simulink model "mcb_pmsm_foc_host_model_dyno"  (R2024b)
settings: Solver=FixedStepDiscrete  StartTime=0.0  StopTime=inf  RelTol=1e-3  EnableMultiTasking=on
values from neighbouring files (symbols this model uses):
  dataType = 'single'    [mcb_pmsm_foc_dyno_f28379d_data.m]
  PU_System_motor1 = mcb_SetPUSystem(pmsm_motor1,inverter_motor1)    [mcb_pmsm_foc_dyno_f28379d_data.m]
  PU_System_motor2 = mcb_SetPUSystem(pmsm_motor2,inverter_motor2)    [mcb_pmsm_foc_dyno_f28379d_data.m]
  Ts = T_pwm    (= 5e-05)    [mcb_pmsm_foc_dyno_f28379d_data.m]
libraries: instrumentseriallib x4, simulink x3
settings Model: Creator=The MathWorks, Inc.  LastModifiedBy=giova
settings SolverCC: AlgebraicLoopSolver=TrustRegion  MaxZcPerStep=1
settings DataIOCC: LimitDataPoints=on  SaveFormat=Array  ReturnWorkspaceOutputs=off
settings OptimizationCC: ReuseModelBlockBuffer=off  LifeSpan=1  EfficientTunableParamExpr=on
settings DebuggingCC: UnderspecifiedInitializationDetection=Classic  MergeDetectMultiDrivingBlocksExec=none  SolverPrmCheckMsg=warning  ParameterPrecisionLossMsg=none  UnconnectedInputMsg=warning  UnconnectedOutputMsg=warning  UnconnectedLineMsg=warning  AllowSymbolicDim=off  PregeneratedLibrarySubsystemCodeDiagnostic=none  SubsystemReferenceDiagnosticForUnitTest=warning  SFUnexpectedBacktrackingDiag=warning  SFNoUnconditionalDefaultTransitionDiag=warning  SFExecutionAtInitializationDiag=none  ArithmeticOperatorsInVariantConditions=warning
settings HardwareCC: ProdBitPerPointer=32  ProdLargestAtomicFloat=None  ProdIntDivRoundTo=Undefined  ProdEndianess=Unspecified  ProdWordSize=32  ProdHWDeviceType=32-bit Generic
settings ModelReferenceCC: EnableRefExpFcnMdlSchedulingChecks=on  PropagateSignalLabelsOutOfModel=off
settings SFSimCC: SimUseLocalCustomCode=off  MATLABDynamicMemAlloc=off
settings RTWCC: Description=Real-Time Workshop Embedded Coder  SystemTargetFile=ert.tlc  TemplateMakefile=ert_default_tmf  GenerateReport=on  RTWUseLocalCustomCode=off  IncludeHyperlinkInReport=on  LaunchReport=on  GenerateTraceInfo=on  GenerateTraceReport=on  GenerateTraceReportSl=on  GenerateTraceReportSf=on  GenerateTraceReportEml=on  GPUComputeCapability=3.5  DLArmComputeVersion=19.05
settings CodeAppCC: IgnoreCustomStorageClasses=off  StateflowObjectComments=on  InternalIdentifier=Classic
settings ERTTargetCC: MultiwordLength=2048  GenerateSampleERTMain=on  InlinedParameterPlacement=Hierarchical  ERTCustomFileTemplate=example_file_process.tlc  ConvertIfToSwitch=off  SuppressUnreachableDefaultCases=off  DynamicArrayContainerType=coder::array
settings ConfigComp: CovMetricSettings=dw  CovSaveCumulativeToWorkspaceVar=on  CovSaveSingleToWorkspaceVar=on  CovExternalEMLEnable=off  CovSFcnEnable=off

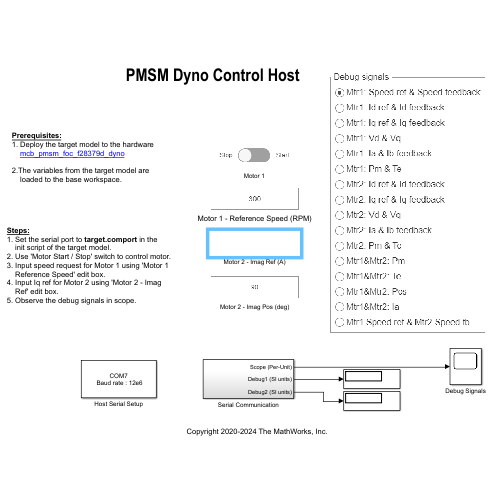
[thumbnail: Simulink's stored preview of the top-level diagram]
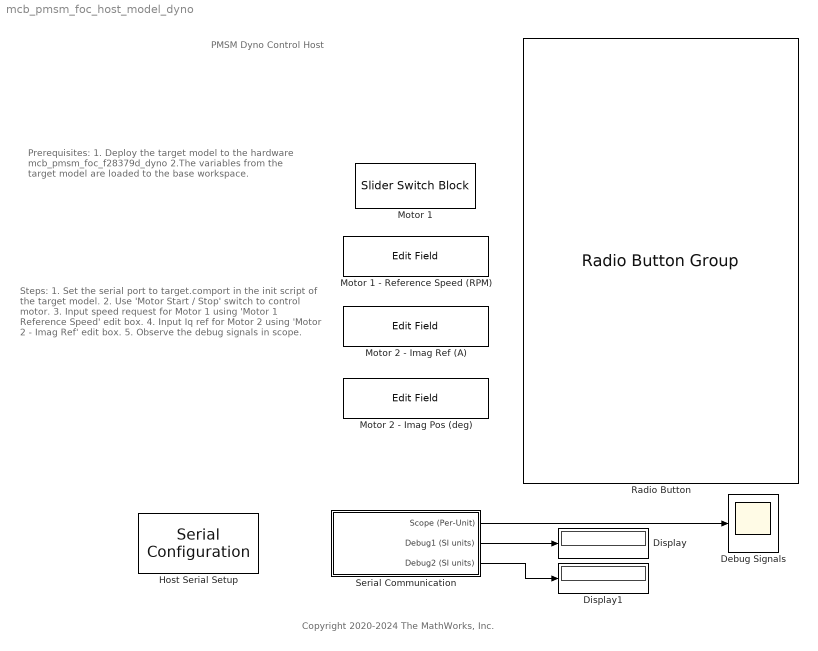
== system mcb_pmsm_foc_host_model_dyno ==
  note: PMSM Dyno Control Host
  note: Copyright 2020-2024 The MathWorks, Inc.
  note: Steps:
      | 1. Set the serial port to target.comport in the
      | init script of the target model.
      | 2. Use 'Motor Start / Stop' switch to control motor.
      | 3. Input speed request for Motor 1 using 'Motor 1
      | Reference Speed' edit box.
      | 4. Input Iq ref for Motor 2 using 'Motor 2 - Imag
      | Ref' edit box.
      | 5. Observe the debug signals in scope.
  note: Prerequisites:
      | 1. Deploy the target model to the hardware
      | mcb_pmsm_foc_f28379d_dyno
      |
      | 2.The variables from the target model are
      | loaded to the base workspace.
  Debug Signals : Scope
  Display : Display
  Display1 : Display
  Host Serial Setup : instrumentseriallib/Serial Configuration  Priority=-99  PortSel=COM7  Port=COM7  ComPort=COM7  BaudRate=12e6  DataBits=8  Parity=none  StopBits=1  ByteOrder=little-endian  FlowControl=none  Timeout=2  SimulateUsing=Interpreted execution  BlockInModel=on  aMode=5
      settings: LibrarySourceBlock=mcblib/Protection and Diagnostics/Host Serial Setup
  Motor 1 : SliderSwitchBlock  LabelPosition=Hide
      settings: Values={{'Stop', 'Start'}, [0 1]}
  Motor 1 - Reference Speed (RPM) : EditField  LabelPosition=Hide  ShowInitialText=on  Alignment=Center
  Motor 2 - Imag Pos (deg) : EditField  LabelPosition=Hide  ShowInitialText=on  Alignment=Center
  Motor 2 - Imag Ref (A) : EditField  LabelPosition=Hide  ShowInitialText=on  Alignment=Center
  Radio Button : RadioButtonGroup  LabelPosition=Hide  SelectedLabel=Mtr1: Speed ref & Speed feedback  ButtonGroupName=Debug signals
      settings: Values={{'Mtr1: Speed ref & Speed feedback', 'Mtr1: Id ref & Id feedback', 'Mtr1: Iq ref & Iq feedback', 'Mtr1: Vd & Vq', 'Mtr1: Ia & Ib feedback', 'Mtr1: Pm & Te', 'Mtr2: Id ref & Id feedback', 'Mtr2: Iq ref & Iq feedback', 'Mtr2: Vd & Vq', 'Mtr2: Ia & Ib feedback', 'Mtr2: Pm & Te', 'Mtr1&Mtr2: Pm', 'Mtr1&Mtr2: Te', 'Mtr1&Mtr2: Pos', 'Mtr1&Mtr2: Ia', 'Mtr1 Speed ref & Mtr2 Speed fb'}, [1 2 3 4 5 6 7 8 9 10 11 12 13 14 15 0]}
  Serial Communication : Subsystem
  wires:
  Serial Communication/1(Scope (Per-Unit)) -> Debug Signals/1
  Serial Communication/2(Debug1 (SI units)) -> Display/1
  Serial Communication/3(Debug2 (SI units)) -> Display1/1

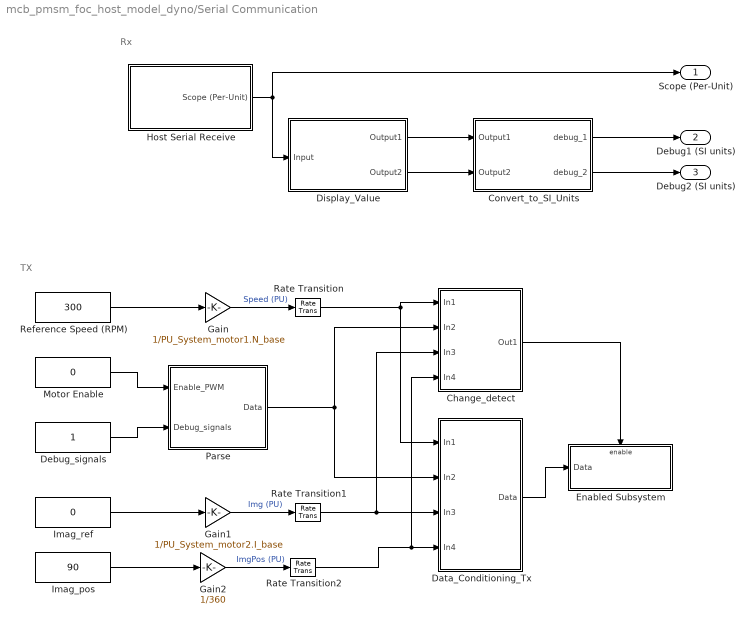
== system mcb_pmsm_foc_host_model_dyno/Serial Communication ==
  note: Rx
  note: TX
  Change_detect : Subsystem
  Convert_to_SI_Units : Subsystem
  Data_Conditioning_Tx : Subsystem  Variant=on
  Debug_signals : Constant  OutDataTypeStr=uint16  SampleTime=0.03
  Display_Value : MATLAB Function  TreatAsAtomicUnit=on
  Enabled Subsystem : Subsystem  TreatAsAtomicUnit=on
  Gain : Gain  Gain=1/PU_System_motor1.N_base  RndMeth=Simplest  OutDataTypeStr=Inherit: Same as input
  Gain1 : Gain  Gain=1/PU_System_motor2.I_base  RndMeth=Simplest  OutDataTypeStr=Inherit: Same as input
  Gain2 : Gain  Gain=1/360  RndMeth=Simplest  OutDataTypeStr=Inherit: Same as input
  Host Serial Receive : Subsystem  Variant=on
  Imag_pos : Constant  Value=90  VectorParams1D=off  OutDataTypeStr=single  SampleTime=0.03
  Imag_ref : Constant  Value=0  VectorParams1D=off  OutDataTypeStr=single  SampleTime=0.03
  Motor Enable : Constant  Value=0  VectorParams1D=off  OutDataTypeStr=uint16  SampleTime=0.03
  Parse : Subsystem
  Rate Transition : RateTransition  OutPortSampleTime=0.03
  Rate Transition1 : RateTransition  OutPortSampleTime=0.03
  Rate Transition2 : RateTransition  OutPortSampleTime=0.03
  Reference Speed (RPM) : Constant  Value=300  VectorParams1D=off  OutDataTypeStr=single  SampleTime=0.03
  Scope (Per-Unit) : Outport
  Debug1 (SI units) : Outport  Port=2
  Debug2 (SI units) : Outport  Port=3
  wires:
  Rate Transition2/1 -> Change_detect/4(In4), Data_Conditioning_Tx/4(In4)
  Imag_pos/1 -> Gain2/1
  Gain2/1 -> Rate Transition2/1  "ImgPos (PU)"
  Gain1/1 -> Rate Transition1/1  "Img (PU)"
  Rate Transition1/1 -> Change_detect/3(In3), Data_Conditioning_Tx/3(In3)
  Imag_ref/1 -> Gain1/1
  Motor Enable/1 -> Parse/1(Enable_PWM)
  Change_detect/1(Out1) -> Enabled Subsystem/Enable
  Reference Speed (RPM)/1 -> Gain/1
  Rate Transition/1 -> Data_Conditioning_Tx/1(In1), Change_detect/1(In1)
  Parse/1(Data) -> Change_detect/2(In2), Data_Conditioning_Tx/2(In2)
  Data_Conditioning_Tx/1(Data) -> Enabled Subsystem/1(Data)
  Gain/1 -> Rate Transition/1  "Speed (PU)"
  Debug_signals/1 -> Parse/2(Debug_signals)
  Convert_to_SI_Units/2(debug_2) -> Debug2 (SI units)/1
  Convert_to_SI_Units/1(debug_1) -> Debug1 (SI units)/1
  Host Serial Receive/1(Scope (Per-Unit)) -> Scope (Per-Unit)/1, Display_Value/1(Input)
  Display_Value/2(Output2) -> Convert_to_SI_Units/2(Output2)
  Display_Value/1(Output1) -> Convert_to_SI_Units/1(Output1)

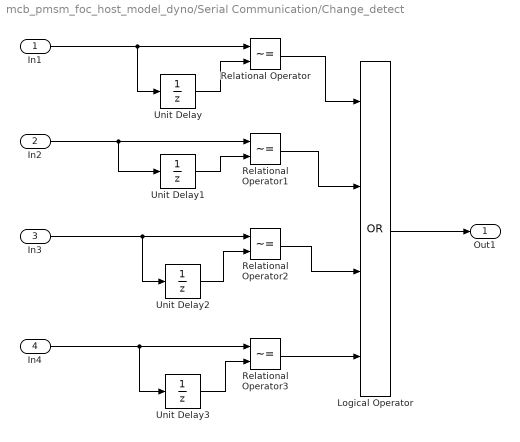
== system mcb_pmsm_foc_host_model_dyno/Serial Communication/Change_detect ==
  In1 : Inport
  In2 : Inport  Port=2
  In3 : Inport  Port=3
  In4 : Inport  Port=4
  Logical Operator : Logic  Operator=OR  Inputs=4  AllPortsSameDT=off  OutDataTypeStr=boolean
  Relational Operator{,1..3} (4 alike) : RelationalOperator  Operator=~=  OutDataTypeStr=boolean  InputSameDT=off
  Unit Delay : UnitDelay  InitialCondition=0.5  SampleTime=-1  HasFrameUpgradeWarning=on
  Unit Delay1 : UnitDelay  SampleTime=-1  HasFrameUpgradeWarning=on
  Unit Delay2 : UnitDelay  InitialCondition=0.5  SampleTime=-1  HasFrameUpgradeWarning=on
  Unit Delay3 : UnitDelay  InitialCondition=0.5  SampleTime=-1  HasFrameUpgradeWarning=on
  Out1 : Outport  VectorParamsAs1DForOutWhenUnconnected=off
  wires:
  In2/1 -> Relational Operator1/1, Unit Delay1/1
  Relational Operator1/1 -> Logical Operator/2
  Unit Delay1/1 -> Relational Operator1/2
  Unit Delay/1 -> Relational Operator/2
  In1/1 -> Unit Delay/1, Relational Operator/1
  Relational Operator/1 -> Logical Operator/1
  Logical Operator/1 -> Out1/1
  Relational Operator2/1 -> Logical Operator/3
  Unit Delay2/1 -> Relational Operator2/2
  In3/1 -> Unit Delay2/1, Relational Operator2/1
  In4/1 -> Unit Delay3/1, Relational Operator3/1
  Unit Delay3/1 -> Relational Operator3/2
  Relational Operator3/1 -> Logical Operator/4

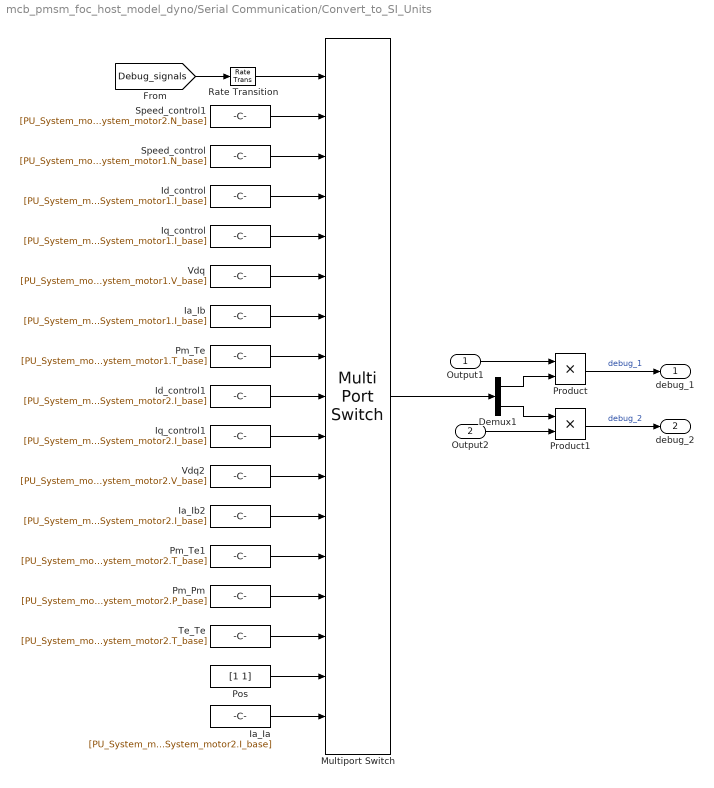
== system mcb_pmsm_foc_host_model_dyno/Serial Communication/Convert_to_SI_Units ==
  Output1 : Inport
  Output2 : Inport  Port=2
  Demux1 : Demux  Outputs=2
  Ia_Ia : Constant  Value=[PU_System_motor1.I_base PU_System_motor2.I_base]  OutDataTypeStr=single  SampleTime=-1
  Ia_Ib : Constant  Value=[PU_System_motor1.I_base PU_System_motor1.I_base]  OutDataTypeStr=single  SampleTime=-1
  Ia_Ib2 : Constant  Value=[PU_System_motor2.I_base PU_System_motor2.I_base]  OutDataTypeStr=single  SampleTime=-1
  Id_control : Constant  Value=[PU_System_motor1.I_base PU_System_motor1.I_base]  OutDataTypeStr=single  SampleTime=-1
  Id_control1 : Constant  Value=[PU_System_motor2.I_base PU_System_motor2.I_base]  OutDataTypeStr=single  SampleTime=-1
  Iq_control : Constant  Value=[PU_System_motor1.I_base PU_System_motor1.I_base]  OutDataTypeStr=single  SampleTime=-1
  Iq_control1 : Constant  Value=[PU_System_motor2.I_base PU_System_motor2.I_base]  OutDataTypeStr=single  SampleTime=-1
  Multiport Switch : MultiPortSwitch  DataPortOrder=Zero-based contiguous  Inputs=16  DiagnosticForDefault=Warning  zeroidx=on  OutDataTypeStr=single  RndMeth=Simplest  SaturateOnIntegerOverflow=off  InputSameDT=off
  Pm_Pm : Constant  Value="[PU_System_motor1.P_base  PU_System_motor2.P_base]"  OutDataTypeStr=single  SampleTime=-1
  Pm_Te : Constant  Value="[PU_System_motor1.P_base  PU_System_motor1.T_base]"  OutDataTypeStr=single  SampleTime=-1
  Pm_Te1 : Constant  Value="[PU_System_motor2.P_base  PU_System_motor2.T_base]"  OutDataTypeStr=single  SampleTime=-1
  Pos : Constant  Value=[1 1]  OutDataTypeStr=single  SampleTime=-1
  Product : Product
  Product1 : Product
  Rate Transition : RateTransition  Deterministic=off
  Speed_control : Constant  Value=[PU_System_motor1.N_base PU_System_motor1.N_base]  OutDataTypeStr=single  SampleTime=-1
  Speed_control1 : Constant  Value=[PU_System_motor1.N_base PU_System_motor2.N_base]  OutDataTypeStr=single  SampleTime=-1
  Te_Te : Constant  Value="[PU_System_motor1.T_base  PU_System_motor2.T_base]"  OutDataTypeStr=single  SampleTime=-1
  Vdq : Constant  Value=[PU_System_motor1.V_base PU_System_motor1.V_base]  OutDataTypeStr=single  SampleTime=-1
  Vdq2 : Constant  Value=[PU_System_motor2.V_base PU_System_motor2.V_base]  OutDataTypeStr=single  SampleTime=-1
  debug_1 : Outport
  debug_2 : Outport  Port=2
  wires:
  Product/1 -> debug_1/1  "debug_1"
  Product1/1 -> debug_2/1  "debug_2"
  [Debug_signals] -> Rate Transition/1
  Multiport Switch/1 -> Demux1/1
  Demux1/1 -> Product/2
  Output1/1 -> Product/1
  Rate Transition/1 -> Multiport Switch/1
  Pos/1 -> Multiport Switch/16
  Ia_Ia/1 -> Multiport Switch/17
  Te_Te/1 -> Multiport Switch/15
  Pm_Pm/1 -> Multiport Switch/14
  Pm_Te1/1 -> Multiport Switch/13
  Ia_Ib2/1 -> Multiport Switch/12
  Vdq2/1 -> Multiport Switch/11
  Iq_control1/1 -> Multiport Switch/10
  Id_control1/1 -> Multiport Switch/9
  Pm_Te/1 -> Multiport Switch/8
  Ia_Ib/1 -> Multiport Switch/7
  Vdq/1 -> Multiport Switch/6
  Iq_control/1 -> Multiport Switch/5
  Id_control/1 -> Multiport Switch/4
  Speed_control/1 -> Multiport Switch/3
  Speed_control1/1 -> Multiport Switch/2
  Demux1/2 -> Product1/1
  Output2/1 -> Product1/2

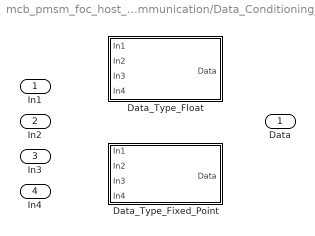
== system mcb_pmsm_foc_host_model_dyno/Serial Communication/Data_Conditioning_Tx ==
  In1 : Inport
  In2 : Inport  Port=2
  In3 : Inport  Port=3
  In4 : Inport  Port=4
  Data_Type_Fixed_Point : Subsystem  VariantControl=~isequal(dataType, 'single')
  Data_Type_Float : Subsystem  VariantControl=isequal(dataType, 'single')
  Data : Outport

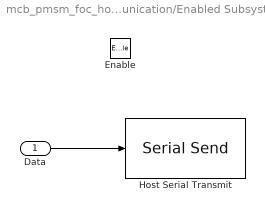
== system mcb_pmsm_foc_host_model_dyno/Serial Communication/Enabled Subsystem ==
  Data : Inport
  Enable : EnablePort
  Host Serial Transmit : instrumentseriallib/Serial Send  PortSel=COM7  Port=COM7  ComPort=COM7  Header=[]  Terminator=<none>  CustomTerminator=[]  EnableBlockingMode=off  SimulateUsing=Interpreted execution  BlockInModel=on  aMode=5
      settings: LibrarySourceBlock=mcblib/Protection and Diagnostics/Host Serial Transmit
  wires:
  Data/1 -> Host Serial Transmit/1

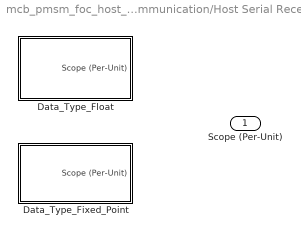
== system mcb_pmsm_foc_host_model_dyno/Serial Communication/Host Serial Receive ==
  Data_Type_Fixed_Point : Subsystem  VariantControl=~isequal(dataType, 'single')
  Data_Type_Float : Subsystem  VariantControl=isequal(dataType, 'single')
  Scope (Per-Unit) : Outport

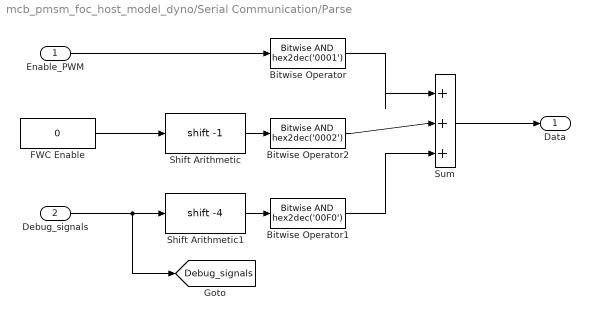
== system mcb_pmsm_foc_host_model_dyno/Serial Communication/Parse ==
  Enable_PWM : Inport
  Debug_signals : Inport  Port=2
  Bitwise Operator : simulink/Logic and Bit Operations/Bitwise Operator  logicop=AND  UseBitMask=on  BitMask=hex2dec('0001')  BitMaskRealWorld=Stored Integer
  Bitwise Operator1 : simulink/Logic and Bit Operations/Bitwise Operator  logicop=AND  UseBitMask=on  BitMask=hex2dec('00F0')  BitMaskRealWorld=Stored Integer
  Bitwise Operator2 : simulink/Logic and Bit Operations/Bitwise Operator  logicop=AND  UseBitMask=on  BitMask=hex2dec('0002')  BitMaskRealWorld=Stored Integer
  FWC Enable : Constant  Value=0  VectorParams1D=off  OutDataTypeStr=uint16  SampleTime=0.03
  Shift Arithmetic : ArithShift  BitShiftNumber=-1
  Shift Arithmetic1 : ArithShift  BitShiftNumber=-4
  Sum : Sum  Inputs=|+++
  Data : Outport
  tag scope: Debug_signals=global
  wires:
  Bitwise Operator/1 -> Sum/1
  Debug_signals/1 -> [Debug_signals], Shift Arithmetic1/1
  Sum/1 -> Data/1
  Shift Arithmetic1/1 -> Bitwise Operator1/1
  Shift Arithmetic/1 -> Bitwise Operator2/1
  Bitwise Operator1/1 -> Sum/3
  FWC Enable/1 -> Shift Arithmetic/1
  Bitwise Operator2/1 -> Sum/2
  Enable_PWM/1 -> Bitwise Operator/1

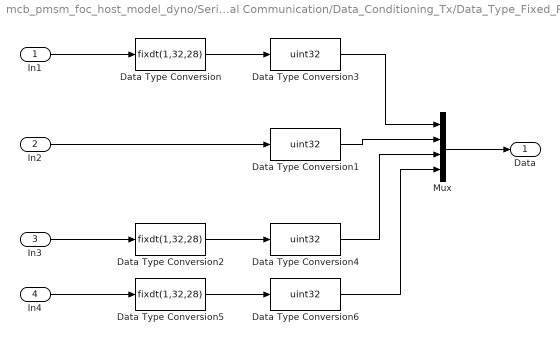
== system mcb_pmsm_foc_host_model_dyno/Serial Communication/Data_Conditioning_Tx/Data_Type_Fixed_Point ==
  In1 : Inport
  In2 : Inport  Port=2
  In3 : Inport  Port=3
  In4 : Inport  Port=4
  Data Type Conversion : DataTypeConversion  OutDataTypeStr=fixdt(1,32,28)  RndMeth=Simplest  SaturateOnIntegerOverflow=off
  Data Type Conversion1 : DataTypeConversion  OutDataTypeStr=uint32  RndMeth=Simplest  SaturateOnIntegerOverflow=off
  Data Type Conversion2 : DataTypeConversion  OutDataTypeStr=fixdt(1,32,28)  RndMeth=Simplest  SaturateOnIntegerOverflow=off
  Data Type Conversion3 : DataTypeConversion  OutDataTypeStr=uint32  ConvertRealWorld=Stored Integer (SI)  RndMeth=Simplest  SaturateOnIntegerOverflow=off
  Data Type Conversion4 : DataTypeConversion  OutDataTypeStr=uint32  ConvertRealWorld=Stored Integer (SI)  RndMeth=Simplest  SaturateOnIntegerOverflow=off
  Data Type Conversion5 : DataTypeConversion  OutDataTypeStr=fixdt(1,32,28)  RndMeth=Simplest  SaturateOnIntegerOverflow=off
  Data Type Conversion6 : DataTypeConversion  OutDataTypeStr=uint32  ConvertRealWorld=Stored Integer (SI)  RndMeth=Simplest  SaturateOnIntegerOverflow=off
  Mux : Mux
  Data : Outport
  wires:
  In1/1 -> Data Type Conversion/1
  Data Type Conversion3/1 -> Mux/1
  Data Type Conversion/1 -> Data Type Conversion3/1
  In2/1 -> Data Type Conversion1/1
  Data Type Conversion1/1 -> Mux/2
  Mux/1 -> Data/1
  Data Type Conversion2/1 -> Data Type Conversion4/1
  Data Type Conversion4/1 -> Mux/3
  In3/1 -> Data Type Conversion2/1
  In4/1 -> Data Type Conversion5/1
  Data Type Conversion5/1 -> Data Type Conversion6/1
  Data Type Conversion6/1 -> Mux/4

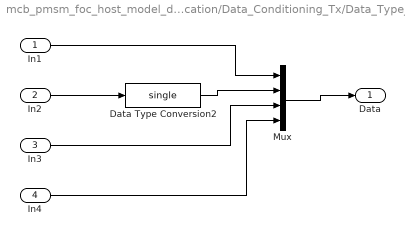
== system mcb_pmsm_foc_host_model_dyno/Serial Communication/Data_Conditioning_Tx/Data_Type_Float ==
  In1 : Inport
  In2 : Inport  Port=2
  In3 : Inport  Port=3
  In4 : Inport  Port=4
  Data Type Conversion2 : DataTypeConversion  OutDataTypeStr=single  RndMeth=Simplest  SaturateOnIntegerOverflow=off
  Mux : Mux
  Data : Outport
  wires:
  In1/1 -> Mux/1
  Mux/1 -> Data/1
  In2/1 -> Data Type Conversion2/1
  Data Type Conversion2/1 -> Mux/2
  In3/1 -> Mux/3
  In4/1 -> Mux/4

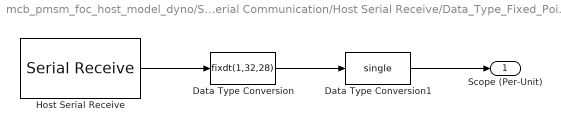
== system mcb_pmsm_foc_host_model_dyno/Serial Communication/Host Serial Receive/Data_Type_Fixed_Point ==
  Data Type Conversion : DataTypeConversion  OutDataTypeStr=fixdt(1,32,28)  ConvertRealWorld=Stored Integer (SI)  RndMeth=Simplest  SaturateOnIntegerOverflow=off
  Data Type Conversion1 : DataTypeConversion  OutDataTypeStr=single  RndMeth=Simplest  SaturateOnIntegerOverflow=off
  Host Serial Receive : instrumentseriallib/Serial Receive  PortSel=target.comport  Port=target.comport  ComPort=target.comport  DataType=uint32  SaveDataType=uint8  ToggleHeader=on  Header='SSSS'  ToggleDataSize=on  DataSize=[600 2]  ToggleTerminator=on  Terminator=Custom terminator  CustomTerminator='EEEE'  InputFormat=Row major  EnableBlockingMode=on  ActionDataUnavailable=Output custom value  ActionWhenDataUnavailable=Output custom value  CustomValue=4  SampleTime=600*Ts  SimulateUsing=Interpreted execution  BlockInModel=on  aMode=5
      settings: LibrarySourceBlock=mcblib/Protection and Diagnostics/Host Serial Receive
  Scope (Per-Unit) : Outport
  wires:
  Data Type Conversion/1 -> Data Type Conversion1/1
  Host Serial Receive/1 -> Data Type Conversion/1
  Data Type Conversion1/1 -> Scope (Per-Unit)/1

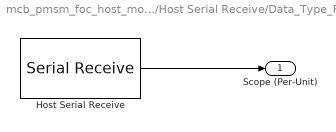
== system mcb_pmsm_foc_host_model_dyno/Serial Communication/Host Serial Receive/Data_Type_Float ==
  Host Serial Receive : instrumentseriallib/Serial Receive  PortSel=COM7  Port=COM7  ComPort=COM7  DataType=single  SaveDataType=uint8  ToggleHeader=on  Header='SSSS'  ToggleDataSize=on  DataSize=[600 2]  ToggleTerminator=on  Terminator=Custom terminator  CustomTerminator='EEEE'  InputFormat=Row major  EnableBlockingMode=on  ActionDataUnavailable=Output custom value  ActionWhenDataUnavailable=Output custom value  CustomValue=4  SampleTime=600*Ts  SimulateUsing=Interpreted execution  BlockInModel=on  aMode=5
      settings: LibrarySourceBlock=mcblib/Protection and Diagnostics/Host Serial Receive
  Scope (Per-Unit) : Outport
  wires:
  Host Serial Receive/1 -> Scope (Per-Unit)/1

== matlab function mcb_pmsm_foc_host_model_dyno/Serial Communication/Display_Value ==
  data: Output1 output; Input input; Output2 output
function [Output1, Output2] = unBuf (Input)
%% ************************************************************************
% Unbuffer function
% Outputs first received serial data from buffer for both signals

% Copyright 2020 The MathWorks, Inc.

selSignal= Input(:, 1);
Output1 = selSignal(1,1);
selSignal = Input(:, 2);
Output2 = selSignal(1,1);
end
